simulink subsystem "Estimator"  (R2025a)
settings: Solver=VariableStepAuto  StartTime=0.0  StopTime=10.0  RelTol=1e-3
undefined symbols (not defined in the file): config
settings Model: Creator=Jackt  LastModifiedBy=Jackt

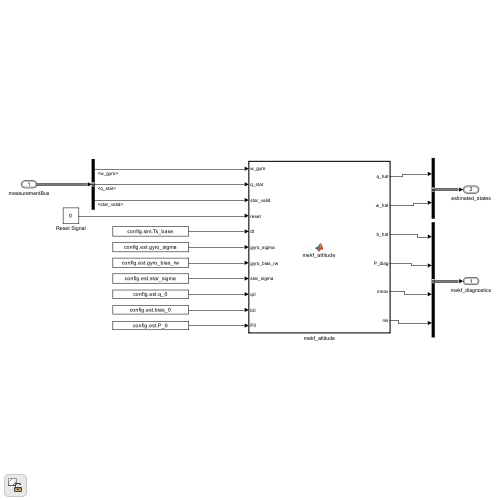
[thumbnail: Simulink's stored preview of the top-level diagram]
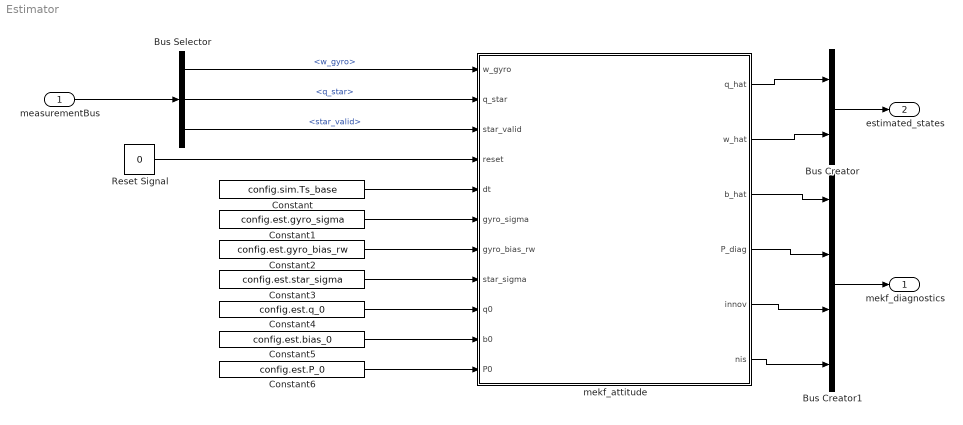
== system Estimator ==
  measurementBus : Inport  OutDataTypeStr=Bus: measurementBus
  Bus Creator : BusCreator  Inputs=2
  Bus Creator1 : BusCreator  Inputs=4
  Bus Selector : BusSelector  OutputSignals=w_gyro,q_star,star_valid
  Constant : Constant  Value=config.sim.Ts_base  VectorParams1D=off
  Constant1 : Constant  Value=config.est.gyro_sigma  VectorParams1D=off
  Constant2 : Constant  Value=config.est.gyro_bias_rw  VectorParams1D=off
  Constant3 : Constant  Value=config.est.star_sigma  VectorParams1D=off
  Constant4 : Constant  Value=config.est.q_0  VectorParams1D=off
  Constant5 : Constant  Value=config.est.bias_0  VectorParams1D=off
  Constant6 : Constant  Value=config.est.P_0  VectorParams1D=off
  Reset Signal : Constant  Value=0
  mekf_attitude : MATLAB Function  TreatAsAtomicUnit=on
  mekf_diagnostics : Outport  OutDataTypeStr=Bus: mekf_diagnostics
  estimated_states : Outport  Port=2  OutDataTypeStr=Bus: estimatedStateBus
  wires:
  mekf_attitude/1(q_hat) -> Bus Creator/1
  mekf_attitude/2(w_hat) -> Bus Creator/2
  mekf_attitude/3(b_hat) -> Bus Creator1/1
  mekf_attitude/4(P_diag) -> Bus Creator1/2
  mekf_attitude/5(innov) -> Bus Creator1/3
  mekf_attitude/6(nis) -> Bus Creator1/4
  Bus Creator1/1 -> mekf_diagnostics/1
  Bus Creator/1 -> estimated_states/1
  Constant6/1 -> mekf_attitude/11(P0)
  Constant5/1 -> mekf_attitude/10(b0)
  Constant4/1 -> mekf_attitude/9(q0)
  Constant3/1 -> mekf_attitude/8(star_sigma)
  Constant2/1 -> mekf_attitude/7(gyro_bias_rw)
  Constant1/1 -> mekf_attitude/6(gyro_sigma)
  Constant/1 -> mekf_attitude/5(dt)
  Reset Signal/1 -> mekf_attitude/4(reset)
  Bus Selector/3 -> mekf_attitude/3(star_valid)  "<star_valid>"
  Bus Selector/2 -> mekf_attitude/2(q_star)  "<q_star>"
  Bus Selector/1 -> mekf_attitude/1(w_gyro)  "<w_gyro>"
  measurementBus/1 -> Bus Selector/1

== matlab function Estimator/mekf_attitude ==
  data: q_hat output; w_hat output; b_hat output; P_diag output; innov output; nis output; w_gyro input; q_star input; star_valid input; reset input; dt input; gyro_sigma input; gyro_bias_rw input; star_sigma input; q0 input; b0 input; P0 input
function [q_hat, w_hat, b_hat, P_diag, innov, nis] = mekf_attitude(w_gyro, q_star, star_valid, reset, dt, gyro_sigma, gyro_bias_rw, star_sigma, q0, b0, P0)
%MEKF_ATTITUDE Multiplicative EKF for attitude (quaternion) and gyro bias (error-state form).
%State (error-state, reset each step): x = [alpha; beta_omega] where
%  alpha      = small-angle attitude error (3x1, rad)
%  beta_omega = gyro bias error (3x1, rad/s)

%Force input shapes
w_gyro = reshape(w_gyro, [3 1]);                 % w_gyro_k      measured body rate (rad/s)
q_star = reshape(q_star, [4 1]);                 % q_star_k      measured attitude (scalar-first), if valid

%Initialize persistent filter states
persistent q_hat_km1 b_omega_hat_km1 P_km1 q_prev is_init
if isempty(is_init) || reset
    q_hat_km1      =  q0(1:4);            % q_hat_{0|0}   nominal attitude estimate (unit quaternion)
    b_omega_hat_km1 = b0(1:3);           % b_omega_{0|0} gyro bias estimate (rad/s)
    P_km1          =  P0(1:6, 1:6);            % P_{0|0} covariance of [alpha; beta_omega]
    q_prev         =  q_hat_km1;     % q_prev        sign-continuity reference
    is_init        =  true;          % is_init       initialization flag
end

%Initialize measurement outputs (reported each call)
innov = zeros(3,1);                              % innov_k       3x1 innovation in rotvec space (rad)
nis   = 0;                                       % nis_k         normalized innovation squared

%Interpret star_valid as "a usable star tracker measurement is available this step"
sv = (star_valid ~= 0);                          % sv_k          0/1 measurement availability

%Build noise covariances
R_k = (star_sigma^2) * eye(3);                   % R_k           star tracker noise in rotvec space (rad^2)
Q_k = 1 * diag([ (gyro_sigma^2)*dt * ones(1,3), ...   % Q_k           discrete process noise for [alpha; beta_omega]
             (gyro_bias_rw^2)*dt * ones(1,3) ]);

%1) Update the orientation estimate with the measured angular velocity (q_{k|k-1})
w_hat_k = w_gyro - b_omega_hat_km1;              % w_hat_k       bias-corrected body rate estimate (rad/s)

dq_prop = rotvec_to_quat(0.5*w_hat_k*dt);        % dq_prop       delta quaternion from gyro integration
q_hat_km1 = quatmultiply_sf(q_hat_km1, dq_prop); % q_hat_{k|k-1} nominal quaternion propagation
q_hat_km1 = q_hat_km1 / max(norm(q_hat_km1), 1e-12); % q_hat_{k|k-1} normalize

%Enforce quaternion sign continuity (prevents sign flips across time)
if dot(q_hat_km1, q_prev) < 0
    q_hat_km1 = -q_hat_km1;                      % q_hat_{k|k-1} sign-aligned
end
q_prev = q_hat_km1;                              % q_prev        update reference

%2) Update the process model (Phi_k = I + F*dt for xdot = F x)
Omega_x = skew(w_hat_k);                         % [w_hat_k x]   skew matrix
F_c = [ -Omega_x, -eye(3);                       % F_c           continuous-time error dynamics for [alpha; beta_omega]
        zeros(3),  zeros(3) ];

Phi_k = eye(6) + F_c*dt;                         % Phi_k         discrete state transition (1st-order)

%3) Update the a priori estimate covariance (P_{k|k-1} = Phi*P*Phi' + Q)
P_km1 = Phi_k * P_km1 * Phi_k.' + Q_k;           % P_{k|k-1}     propagate covariance
P_km1 = 0.5*(P_km1 + P_km1.');                   % P symmetry    enforce symmetric covariance

%If no star tracker measurement, stop here: MEKF still outputs q_hat and w_hat each step (gyro-only propagation)
if sv && all(isfinite(q_star)) && (norm(q_star) > 1e-12)

    %Normalize q_star only if used
    q_star = q_star / max(norm(q_star), 1e-12);  % q_star_k      normalize measurement

    %Align measurement sign with estimate (same physical rotation, consistent sign)
    if dot(q_star, q_hat_km1) < 0
        q_star = -q_star;                        % q_star_k      sign-aligned to estimate
    end

    %4) Measurement innovation (y_k) in rotvec space using q_e = inv(q_hat_{k|k-1}) ⊗ q_star
    q_hat_inv = [q_hat_km1(1); -q_hat_km1(2:4)]; % inv(q_hat)    quaternion inverse for unit quaternion
    q_e = quatmultiply_sf(q_hat_inv, q_star);    % q_e           right-invariant error quaternion
    q_e = q_e / max(norm(q_e), 1e-12);           % q_e           normalize

    if q_e(1) < 0
        q_e = -q_e;                              % q_e           shortest-rotation convention
    end

    y_k = quat_log_sf(q_e);                      % y_k           innovation (approx alpha + noise), rad
    innov = y_k;                                 % innov_k       output innovation

    %5) Kalman gain (K_k = P H' (H P H' + R)^{-1})
    H_k = [eye(3), zeros(3)];                    % H_k           measurement Jacobian for attitude-only observation
    S_k = H_k * P_km1 * H_k.' + R_k;             % S_k           innovation covariance
    K_k = (P_km1 * H_k.') / S_k;                 % K_k           Kalman gain

    %6) Update the a posteriori state estimate and covariance
    x_k = K_k * y_k;                             % x_{k|k}       estimated error-state correction [alpha; beta_omega]
    alpha_hat_k = x_k(1:3);                      % alpha_hat_k   attitude error correction (rad)
    db_omega_k  = x_k(4:6);                      % db_omega_k    gyro bias correction (rad/s)

    I6 = eye(6);                                 % I6            identity
    P_km1 = (I6 - K_k*H_k) * P_km1 * (I6 - K_k*H_k).' + K_k*R_k*K_k.'; % Joseph form
    P_km1 = 0.5*(P_km1 + P_km1.');               % P symmetry    enforce symmetric covariance

    %7) Update the a posteriori orientation estimate (q_{k|k} = q_{k|k-1} ⊗ delta_q(alpha))
    b_omega_hat_km1 = b_omega_hat_km1 + db_omega_k; % b_omega_{k|k} bias injection

    dq_inj = rotvec_to_quat(0.5*alpha_hat_k);    % delta_q       error quaternion from small-angle correction
    q_hat_km1 = quatmultiply_sf(q_hat_km1, dq_inj); % q_hat_{k|k}  apply correction
    q_hat_km1 = q_hat_km1 / max(norm(q_hat_km1), 1e-12); % q_hat_{k|k} normalize

    %Enforce quaternion sign continuity after update
    if dot(q_hat_km1, q_prev) < 0
        q_hat_km1 = -q_hat_km1;                  % q_hat_{k|k}   sign-aligned
    end
    q_prev = q_hat_km1;                          % q_prev        update reference

    %Compute normalized innovation squared
    nis = y_k.' * (S_k \ y_k);                   % nis_k         y' S^{-1} y
end

%Package estimator outputs (always produced, even with gyro-only propagation)
q_hat  = q_hat_km1;                              % q_hat         nominal attitude estimate (unit quaternion)
b_hat  = b_omega_hat_km1;                        % b_hat         gyro bias estimate (rad/s)
w_hat  = w_gyro - b_omega_hat_km1;               % w_hat         bias-corrected body rate estimate (rad/s)
P_diag = diag(P_km1);                            % P_diag        diagonal of covariance (6x1)

%Format for Simulink Processing
q_hat =  reshape(q_hat, [4 1]);
b_hat =  reshape(b_hat, [3 1]);
w_hat =  reshape(w_hat, [3 1]);
P_diag = reshape(P_diag, [6 1]);
innov =  reshape(innov, [3 1]);
nis =    double(nis(1));

end

function S = skew(w)
%SKEW Returns the skew-symmetric matrix such that skew(w)*v = w x v.
S = [   0   -w(3)  w(2);
      w(3)    0   -w(1);
     -w(2)  w(1)    0  ];
end

function q = rotvec_to_quat(v)
%ROTVEC_TO_QUAT Converts a half-angle rotation vector v = (theta/2) * u to a unit quaternion.
theta = norm(v);                                 % theta         half-angle magnitude (rad)
if theta < 1e-12
    q = [1; 0; 0; 0];                             % q            identity quaternion
else
    u = v/theta;                                  % u            rotation axis
    q = [cos(theta); u*sin(theta)];               % q            scalar-first quaternion
end
end

function r = quat_log_sf(q)
%QUAT_LOG_SF Log-map from unit quaternion (scalar-first) to rotation vector (full angle).
q = q / max(norm(q), 1e-12);                      % q            normalize
if q(1) < 0
    q = -q;                                       % q            shortest rotation
end
w = max(-1, min(1, q(1)));                        % w            clamp scalar
v = q(2:4);                                       % v            vector part
nv = norm(v);                                     % nv           vector norm
if nv < 1e-8
    r = 2*v;                                      % r            small-angle limit (rad)
else
    ang = 2*atan2(nv, w);                         % ang          full rotation angle (rad)
    r = (ang/nv) * v;                             % r            rotation vector (rad)
end
end

function q = quatmultiply_sf(a, b)
%QUATMULTIPLY_SF Hamilton quaternion multiply (scalar-first): q = a ⊗ b.
w1 = a(1); x1 = a(2); y1 = a(3); z1 = a(4);       % a components
w2 = b(1); x2 = b(2); y2 = b(3); z2 = b(4);       % b components
q = [ w1*w2 - x1*x2 - y1*y2 - z1*z2;
      w1*x2 + x1*w2 + y1*z2 - z1*y2;
      w1*y2 - x1*z2 + y1*w2 + z1*x2;
      w1*z2 + x1*y2 - y1*x2 + z1*w2 ];
end
